simulink model "p3"  (R2021a)
settings: Solver=FixedStepAuto  StartTime=0.0  StopTime=15  RelTol=1e-3
undefined symbols (not defined in the file): sigbuilder_block
settings Model: EnablePacing=on  Creator=Abbas  LastModifiedBy=Abbas

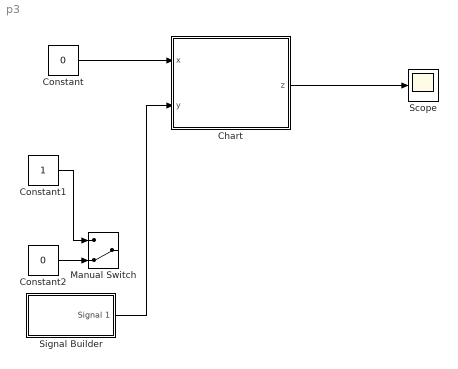
== system p3 ==
  Chart : Stateflow chart  TreatAsAtomicUnit=on
  Constant : Constant  Value=0
  Constant1 : Constant
  Constant2 : Constant  Value=0
  Manual Switch : ManualSwitch  CurrentSetting=0
  Scope : Scope
  Signal Builder : Subsystem  Tag=STV Subsys  LoadFcn=sigbuilder_block('load');  StartFcn=sigbuilder_block('start');  StopFcn=sigbuilder_block('stop');  ClipboardFcn=sigbuilder_block('clipboard');  mask(Sigbuilder block){tuvar=[0:10]}
      mask help: Simulink:masks:SigbuilderBlock_MD
      mask init:
      | if ~strcmp(get_param(bdroot(gcbh),'SimulationStatus'),'stopped') tuvar = sigbuilder_block('maskInit'); end
      settings: CopyFcn=sigbuilder_block('copy');  DeleteFcn=sigbuilder_block('delete');  ModelCloseFcn=sigbuilder_block('modelClose');  PreSaveFcn=sigbuilder_block('preSave');  PauseFcn=sigbuilder_block('pause');  ContinueFcn=sigbuilder_block('continue');  NameChangeFcn=sigbuilder_block('namechange');  OpenFcn=sigbuilder_block('open',[479 849.5 543.5 239 ]);  CloseFcn=sigbuilder_block('close');
      mask Display: plot(0, 0, 100, 100,[2, 2, 32, 32, 2], [68, 8, 8, 68, 68],[32, 2], [38, 38], [32, 19, 2],[53, 60, 44], [32, 17, 17, 2],[16, 16, 31, 31]);txt = getActiveGroup(gcbh);text(2, 100, txt,'verticalAlignment', 'top');
  wires:
  Constant/1 -> Chart/1(x)
  Chart/1(z) -> Scope/1
  Signal Builder/1(Signal 1) -> Chart/2(y)
  Constant1/1 -> Manual Switch/1
  Constant2/1 -> Manual Switch/2

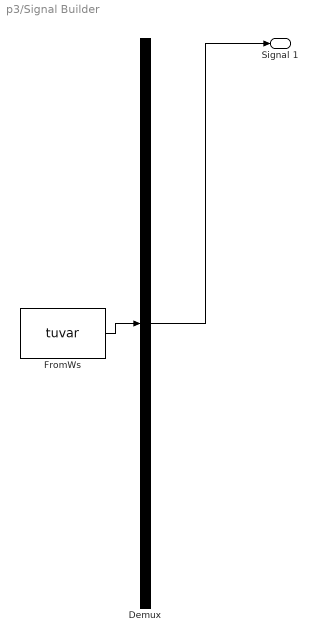
== system p3/Signal Builder ==
  Demux : Demux  Tag=STV Demux  Outputs=1
      settings: DisplayOption=none
  FromWs : FromWorkspace  Tag=STV FromWs  VariableName=tuvar
      SigBuilderData=|
      | common.afterFinalStr = 'Extrapolate'
      | common.sampleTime = 0
      | dataSet.timeRange = [0 10]
      | dataSet.name = 'Group 1'
      | sbobj.Groups.Name = 'Group 1'
      | sbobj.Groups.Signals.Name = 'Signal 1'
      | sbobj.Groups.Signals.XData = [0 7.5 7.5 9 9 10]
      | sbobj.Groups.Signals.YData = [0 0 1 1 0 0]
  Signal 1 : Outport  Tag=STV Outport
  wires:
  Demux/1 -> Signal 1/1
  FromWs/1 -> Demux/1

== stateflow chart p3/Chart ==
  settings: updateMethod=CONTINUOUS
  state FIRST
    du:
    timer1_dot = 1;
  state SECOND
    du:
    timer2_dot = 1;
    timer1_dot = 1;
  state THIRD
    du:
    timer1_dot = 1;
    timer2_dot = 1;
  (default) -> FIRST [order 1]
  (default) -> SECOND [order 2]
  FIRST -> SECOND : [timer1 >= t1 & x == 1]{timer2 = 0 ;}
  SECOND -> FIRST [order 1] : [((timer1>t1+5)|(timer1<t1+2)) & y == 1 ]{timer1=0; timer2 = 0; }
  THIRD -> FIRST [order 1] : [(timer1>timer1_save + 6)]{z = 0 ;}
  SECOND -> THIRD [order 2] : [((timer1<=t1+5) & (timer1>=t1+2)) & y == 1 & timer2>=t2 ]{timer1_save = timer1 ; timer2_save = timer2}
  THIRD -> THIRD [order 2] : [(timer1<=timer1_save + 6) & (timer2>=timer2_save+1)]{z =1}
  data: timer1 local =0; x input; timer2 local =0; y input; t1 local =5; t2 local =2; z output; timer1_save local; timer2_save local
  data timer1 settings: updateMethod=SF_CONTINUOUS_TIME_DATA
  data timer2 settings: updateMethod=SF_CONTINUOUS_TIME_DATA
